simulink model "FullModel_Slow"  (R2024b)
settings: Solver=VariableStepAuto  StartTime=0.0  StopTime=50  FixedStep=1e-4  RelTol=1e-3  EnableMultiTasking=on
model workspace (MAT data in the model file):
  pidSample = 0.0005
  pwmFreq = 5000
libraries: nesl_utility x15, fl_lib x9, ee_lib x5, slpidlib x2, eeTransforms x1
settings Model: SimulationMode=accelerator  Creator=luigi  LastModifiedBy=luigi
settings SolverCC: AllowMultiTaskInputOutput=on  ConcurrentTasks=on  AutoInsertRateTranBlk=on  EnableFixedStepZeroCrossing=on
settings HardwareCC: ProdBitPerLong=64  ProdLargestAtomicFloat=None  ProdHWDeviceType=AMD->Athlon 64
settings SFSimCC: SimTargetLang=C++
settings RTWCC: RTWVerbose=off

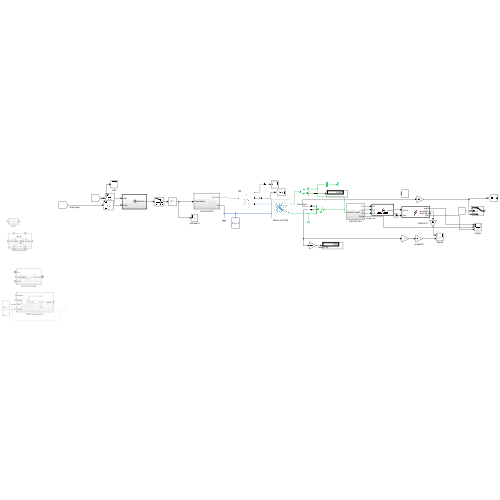
[thumbnail: Simulink's stored preview of the top-level diagram]
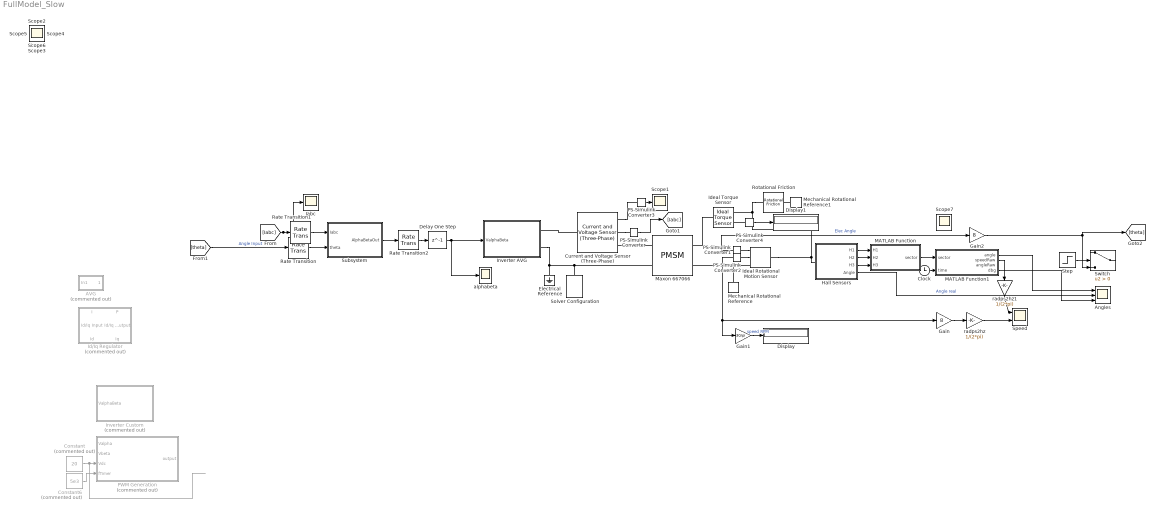
== system FullModel_Slow ==
  AVG : Subsystem  Commented=on
  Angles : Scope  NumInputPorts=3
  Clock : Clock
  Constant : Constant  Commented=on  Value=20
  Constant6 : Constant  Commented=on  Value=5e3
  Current and Voltage Sensor (Three-Phase) : ee_lib/Sensors & Transducers/Current and Voltage Sensor (Three-Phase)  vMeasurementType=ee.enum.vmeasurement.ll  outputUnit=ee.enum.unit.si  SRated=100e6 A*V  VRated=24e3 V  I_specify=off  I_priority=None  I=[0, 0, 0] A  I_nominal_specify=off  I_nominal_value=1  I_nominal_unit=A  V_specify=off  V_priority=None  V=[0, 0, 0] V  V_nominal_specify=off  V_nominal_value=1  V_nominal_unit=V
      settings: InternalSimscapePortConfiguration="{\"Bottom\":[],\"Left\":[{\"id\":\"N1\",\"label\":\"~1\",\"type\":\"foundation.electrical.three_phase\"}],\"Right\":[{\"id\":\"V_output\",\"label\":\"V\",\"type\":\"output\"},{\"id\":\"I_output\",\"label\":\"I\",\"type\":\"output\"},{\"id\":\"N2\",\"label\":\"~2\",\"type\":\"foundation.electrical.three_phase\"}],\"Top\":[]}"
  Delay One Step : Delay  DelayLength=1
  Display : Display
  Display1 : Display
  Electrical Reference : fl_lib/Electrical/Electrical Elements/Electrical Reference
  Gain : Gain  Gain=8
  Gain1 : Gain  Gain=30/pi
  Gain2 : Gain  Gain=8
  Hall Sensors : Subsystem
  Iabc : Scope
  Id/Iq Regulator : Subsystem  Commented=on
      settings: PortSchema="{\"entries\":[{\"content\":{\"sides\":[{\"content\":{\"connectorIds\":[\"In1\"]},\"type\":\"ConnectorPlacement.EquallySpacedRectSide\",\"uuid\":\"43b3a311-7cb7-4eab-a35c-85d0ca0e3076\"},{\"content\":{\"connectorIds\":[\"Out1\"],\"side\":\"RIGHT\"},\"type\":\"ConnectorPlacement.EquallySpacedRectSide\",\"uuid\":\"ca56bbca-54ba-4ca6-9209-c2819f440ab7\"},{\"content\":{\"connectorIds\":[\"In2\",\"In3\"],\"side\":\"TOP\"},\"type\":\"ConnectorPlacement.EquallySpacedRectSide\",\"uuid\":\"c57e1d45-56ff-40ef-8d87-b012e39b3f70\"},{\"content\":{\"connectorIds\":[\"In4\",\"In5\"],\"side\":\"BOTTOM\"},\"type\":\"ConnectorPlacement.EquallySpacedRectSide\",\"uuid\":\"5c883e63-5688-4569-9eaa-37faa042d8a8\"}]},\"type\":\"ConnectorPlacement.EquallySpacedConnector\",\"uuid\":\"9c051708-b157-4ef2-9fb2-e90e892a94b0\"}],\"packageUris\":[\"http://schema.mathworks.com/mf0/Connector/R2020b\"],\"version\":\"1.0\"}"
  Ideal Rotational Motion Sensor : fl_lib/Mechanical/Mechanical Sensors/Ideal Rotational Motion Sensor  reference=foundation.enum.MeasurementReference.difference  acceleration_port=false  velocity_port=true  position_port=true  wrap_angle=true  offset=0 rad
  Ideal Torque Sensor : fl_lib/Mechanical/Mechanical Sensors/Ideal Torque Sensor
  Inverter AVG : Subsystem
      settings: MinAlgLoopOccurrences=on
  Inverter Custom : Subsystem  Commented=on
      settings: PortSchema="{\"entries\":[{\"content\":{\"sides\":[{\"content\":{\"connectorIds\":[\"LConn1\",\"In1\",\"LConn2\"]},\"type\":\"ConnectorPlacement.EquallySpacedRectSide\",\"uuid\":\"8f29009c-fde7-40c5-b267-68669c6fe162\"},{\"content\":{\"connectorIds\":[\"RConn1\"],\"side\":\"RIGHT\"},\"type\":\"ConnectorPlacement.EquallySpacedRectSide\",\"uuid\":\"42ee2bc7-4e72-4e66-b818-79789fabddd4\"},{\"content\":{\"side\":\"TOP\"},\"type\":\"ConnectorPlacement.EquallySpacedRectSide\",\"uuid\":\"30675e7c-1db2-4723-9999-8a6d31f0d3a7\"}]},\"type\":\"ConnectorPlacement.EquallySpacedConnector\",\"uuid\":\"6307069a-32f5-4400-962e-81599f3d1bde\"}],\"packageUris\":[\"http://schema.mathworks.com/mf0/Connector/R2020b\"],\"version\":\"1.0\"}"
  MATLAB Function : MATLAB Function  TreatAsAtomicUnit=on  SystemSampleTime=0
  MATLAB Function1 : MATLAB Function  TreatAsAtomicUnit=on  SystemSampleTime=1e-4
  Maxon 667066 : ee_lib/Electromechanical/Permanent Magnet/PMSM  port_option=ee.enum.threePhasePort.composite  winding_type=ee.enum.electromech.statorconfiguration.wye  machine_param=ee.enum.pmsm.parameterization.constant  nPolePairs=8  pmflux_param=ee.enum.pmflux.torqueconstant  pm_flux_linkage=0.03 Wb  torque_constant=68 m*mN/A  back_emf_constant=0.18 V*s/rad  stator_param=ee.enum.statorparam.LsLmMs  Ld=0.00019 H  Lq=0.00025 H  idVec=[-200, 0, 200] A  iqVec=[-200, 0, 200] A  LdMatrix=0.0002 * ones(3, 3) H  LqMatrix=0.0002 * ones(3, 3) H  PmMatrix=0.1 * ones(3, 3) Wb  ktMatrix=0.18 * ones(3, 3) N*m/A  keMatrix=0.18 * ones(3, 3) V*s/rad  L0=0.00016 H  Ls=0.261/2 mH  Lm=0 H  Ms=0.261/4 mH  Rs=0.155/2 Ohm  zero_sequence=ee.enum.park.zerosequence.include  axes_param=ee.enum.rotorangle.daxis  loss_param=ee.enum.ironloss.none  losses_oc=[0, 0, 0] W  losses_sc=[0, 0, 0] W  f_losses=60 Hz  Isc_losses=95 A  J=0.01 kg*m^2  lam=0 N*m*s/rad  i_d_specify=off  i_d_priority=None  i_d=0 A  i_d_nominal_specify=off  i_d_nominal_value=1  i_d_nominal_unit=A  i_q_specify=off  i_q_priority=None  i_q=0 A  i_q_nominal_specify=off  i_q_nominal_value=1  i_q_nominal_unit=A  torque_specify=off  torque_priority=None  torque=0 N*m  torque_nominal_specify=off  torque_nominal_value=1  torque_nominal_unit=N*m  angular_velocity_specify=off  angular_velocity_priority=High  angular_velocity=500 rpm  angular_velocity_nominal_specify=off  angular_velocity_nominal_value=1  angular_velocity_nominal_unit=rpm  angular_position_specify=off  angular_position_priority=High  angular_position=0 deg  angular_position_nominal_specify=off  angular_position_nominal_value=1  angular_position_nominal_unit=deg  alpha=3.93e-3 1/K  alpha_flux=-0.001 1/K  Tmeas=298.15 K  stator_thermal_mass=100 J/K  rotor_thermal_mass=200 J/K  Rm_percent_rotor=90  Rd_percent_rotor=30  temperatureA_specify=off  temperatureA_priority=High  temperatureA=25 degC  temperatureA_nominal_specify=off  temperatureA_nominal_value=1  temperatureA_nominal_unit=degC  temperatureB_specify=off  temperatureB_priority=High  temperatureB=25 degC  temperatureB_nominal_specify=off  temperatureB_nominal_value=1  temperatureB_nominal_unit=degC  temperatureC_specify=off  temperatureC_priority=High  temperatureC=25 degC  temperatureC_nominal_specify=off  temperatureC_nominal_value=1  temperatureC_nominal_unit=degC  temperatureR_specify=off  temperatureR_priority=High  temperatureR=25 degC  temperatureR_nominal_specify=off  temperatureR_nominal_value=1  temperatureR_nominal_unit=degC
      settings: InternalSimscapePortConfiguration="{\"Bottom\":[],\"Left\":[{\"id\":\"N\",\"label\":\"~\",\"type\":\"foundation.electrical.three_phase\"},{\"id\":\"n\",\"label\":\"n\",\"type\":\"foundation.electrical.electrical\"}],\"Right\":[{\"id\":\"R\",\"label\":\"R\",\"type\":\"foundation.mechanical.rotational.rotational\"},{\"id\":\"C\",\"label\":\"C\",\"type\":\"foundation.mechanical.rotational.rotational\"}],\"Top\":[]}"
  Mechanical Rotational Reference : fl_lib/Mechanical/Rotational Elements/Mechanical Rotational Reference
  Mechanical Rotational Reference1 : fl_lib/Mechanical/Rotational Elements/Mechanical Rotational Reference
  PS-Simulink Converter{,1..4} (5 alike) : nesl_utility/PS-Simulink Converter  PhysicalDomain=network_engine_domain  SubClassName=ps_output  LeftPortType=input  RightPortType=output  PseudoPeriodic=off  Frequencies=[]  VectorFormat=inherit  Unit=inherit  AffineConversion=off
  PWM Generation : Subsystem  Commented=on
  Rate Transition : RateTransition
  Rate Transition1 : RateTransition
  Rate Transition2 : RateTransition
  Rotational Friction : fl_lib/Mechanical/Rotational Elements/Rotational Friction  brkwy_trq=0.1 N*m  brkwy_vel=0.1 rad/s  Col_trq=0.05 N*m  visc_coef=0.0005 N*m*s/rad  w_specify=off  w_priority=None  w=0 rad/s  w_nominal_specify=off  w_nominal_value=1  w_nominal_unit=rad/s  t_specify=off  t_priority=None  t=0 N*m  t_nominal_specify=off  t_nominal_value=1  t_nominal_unit=N*m
  Scope{,1..7} (8 alike) : Scope
  Solver Configuration : nesl_utility/Solver Configuration  PhysicalDomain=network_engine_domain  SubClassName=solver  LeftPortType=input  RightPortType=generic  Tones=[]  Harmonics=[]  SimulateNoise=off  Profile=off  UseLocalSampling=off  EnableSwitchedLinearOptims=on  FrequencyDomain=off  UseCCode=off  RelTol=0.001  AbsTol=0.001  MinStep=1e-09  ToWorkspace=off  RevertToSquareIcSolve=off  NumHomotopyIterations=100  PhasorMode=off  PhasorModeNumHarmonics=1  ConsistencySolver=NEWTON_XTOL_AFTER_FTOL  IndexReductionMethod=DerivativeReplacement  DoDC=off  ResidualTolerance=1e-09  ConsistencyTolSource=GLOBAL  ConsistencyAbsTol=0.001  ConsistencyRelTol=0.001  ConsistencyTolFactor=0.001  UseLocalSolver=on  LocalSolverChoice=NE_TRAPEZOIDAL_ADVANCER  ResolveIndetEquations=off  FunctionEvalNumThread=1  LocalSolverSampleTime=0.0001  DoFixedCost=off  MaxNonlinIter=3  MaxModeIter=2  ComputeImpulses=off  ImpulseIterations=2  LinearAlgebra=auto  LinearAlgebraNumThread=0  EquationFormulation=NE_TIME_EF  DelaysMemoryBudget=1024  AutomaticFiltering=off  FilteringTimeConstant=0.001  PartitionStorageMethod=AS_NEEDED  PartitionMemoryBudget=1024  PartitionMethod=ROBUST  MultibodyUseLocalSolver=off  MultibodyLocalSolverChoice=ODE1  MultibodyLocalSolverSampleTime=0.001
  Speed : Scope  NumInputPorts=2
  Step : Step  After=2  SampleTime=0
  Subsystem : Subsystem  TreatAsAtomicUnit=on  SystemSampleTime=1e-4
  Switch : Switch  Criteria=u2 > Threshold  SaturateOnIntegerOverflow=off  InputSameDT=off
  alphabeta : Scope
  radps2hz : Gain  Gain=1/(2*pi)
  radps2hz1 : Gain  Gain=1/(2*pi)
  wires:
  PS-Simulink Converter/1 -> [Iabc]
  Delay One Step/1 -> alphabeta/1, Inverter AVG/1(ValphaBeta)
  Hall Sensors/1(H1) -> MATLAB Function/1(H1)
  Hall Sensors/2(H2) -> MATLAB Function/2(H2)
  Hall Sensors/3(H3) -> MATLAB Function/3(H3)
  PS-Simulink Converter2/1 -> Gain1/1, Gain/1
  Constant/1 -> PWM Generation/3(Vdc)
  Constant6/1 -> PWM Generation/4(fTimer)
  PS-Simulink Converter3/1 -> Scope1/1
  Subsystem/1(AlphaBetaOut) -> Rate Transition2/1
  [Iabc] -> Iabc/1, Rate Transition1/1
  Rate Transition/1 -> Subsystem/2(theta)
  Rate Transition1/1 -> Subsystem/1(Iabc)
  Rate Transition2/1 -> Delay One Step/1
  [theta] -> Rate Transition/1  "Angle Input"
  Gain1/1 -> Display/1  "speed RPM"
  Step/1 -> Switch/2
  PS-Simulink Converter4/1 -> Display1/1
  PS-Simulink Converter1/1 -> Gain2/1  "Elec Angle"
  Gain2/1 -> Switch/3, [theta]
  MATLAB Function/1(sector) -> MATLAB Function1/1(sector)
  MATLAB Function1/2(speedRaw) -> radps2hz1/1
  MATLAB Function1/1(angle) -> Angles/1
  Hall Sensors/4(Angle) -> Angles/2  "Angle real"
  MATLAB Function1/4(dbg) -> Angles/3
  Clock/1 -> MATLAB Function1/2(time)
  Gain/1 -> radps2hz/1
  radps2hz/1 -> Speed/2
  radps2hz1/1 -> Speed/1
  connections:
  Solver Configuration/RConn1 -- Inverter AVG/RConn2 -- Electrical Reference/LConn1 -- Maxon 667066/LConn2
  Mechanical Rotational Reference/LConn1 -- Ideal Rotational Motion Sensor/RConn1 -- Maxon 667066/RConn2
  Current and Voltage Sensor (Three-Phase)/RConn3 -- Maxon 667066/LConn1
  PS-Simulink Converter1/LConn1 -- Ideal Rotational Motion Sensor/RConn3
  PS-Simulink Converter2/LConn1 -- Ideal Rotational Motion Sensor/RConn2
  Current and Voltage Sensor (Three-Phase)/RConn2 -- PS-Simulink Converter/LConn1
  Current and Voltage Sensor (Three-Phase)/RConn1 -- PS-Simulink Converter3/LConn1
  Current and Voltage Sensor (Three-Phase)/LConn1 -- Inverter AVG/RConn1
  Mechanical Rotational Reference1/LConn1 -- Rotational Friction/RConn1
  Rotational Friction/LConn1 -- Ideal Rotational Motion Sensor/LConn1 -- Hall Sensors/LConn1 -- Ideal Torque Sensor/RConn1
  Ideal Torque Sensor/LConn1 -- Maxon 667066/RConn1
  PS-Simulink Converter4/LConn1 -- Ideal Torque Sensor/RConn2

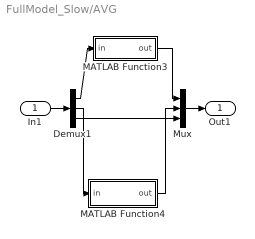
== system FullModel_Slow/AVG ==
  In1 : Inport
  Demux1 : Demux  Outputs=3
  MATLAB Function3 : MATLAB Function  TreatAsAtomicUnit=on  SystemSampleTime=0
  MATLAB Function4 : MATLAB Function  TreatAsAtomicUnit=on  SystemSampleTime=0
  Mux : Mux  Inputs=3
  Out1 : Outport
  wires:
  Demux1/1 -> MATLAB Function3/1(in)
  Demux1/2 -> MATLAB Function4/1(in)
  Demux1/3 -> Mux/3
  In1/1 -> Demux1/1
  MATLAB Function3/1(out) -> Mux/1
  MATLAB Function4/1(out) -> Mux/2
  Mux/1 -> Out1/1

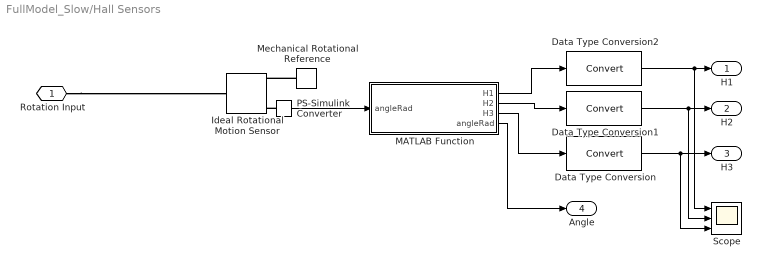
== system FullModel_Slow/Hall Sensors ==
  Data Type Conversion : DataTypeConversion  SaturateOnIntegerOverflow=off  RndMeth=Floor
  Data Type Conversion1 : DataTypeConversion  SaturateOnIntegerOverflow=off  RndMeth=Floor
  Data Type Conversion2 : DataTypeConversion  SaturateOnIntegerOverflow=off  RndMeth=Floor
  Ideal Rotational Motion Sensor : fl_lib/Mechanical/Mechanical Sensors/Ideal Rotational Motion Sensor  reference=foundation.enum.MeasurementReference.difference  acceleration_port=false  velocity_port=true  position_port=true  wrap_angle=true  offset=0 rad
  MATLAB Function : MATLAB Function  TreatAsAtomicUnit=on  SystemSampleTime=0
  Mechanical Rotational Reference : fl_lib/Mechanical/Rotational Elements/Mechanical Rotational Reference
  PS-Simulink Converter : nesl_utility/PS-Simulink Converter  PhysicalDomain=network_engine_domain  SubClassName=ps_output  LeftPortType=input  RightPortType=output  PseudoPeriodic=off  Frequencies=[]  VectorFormat=inherit  Unit=inherit  AffineConversion=off
  Scope : Scope  NumInputPorts=3
  Rotation Input : PMIOPort  Side=Left
  H1 : Outport  OutDataTypeStr=uint8
  H2 : Outport  Port=2  OutDataTypeStr=uint8
  H3 : Outport  Port=3  OutDataTypeStr=uint8
  Angle : Outport  Port=4  OutDataTypeStr=double
  wires:
  MATLAB Function/2(H2) -> Data Type Conversion1/1
  MATLAB Function/3(H3) -> Data Type Conversion/1
  PS-Simulink Converter/1 -> MATLAB Function/1("angleRad ")
  MATLAB Function/1(H1) -> Data Type Conversion2/1
  Data Type Conversion/1 -> Scope/3, H3/1
  Data Type Conversion1/1 -> Scope/2, H2/1
  Data Type Conversion2/1 -> H1/1, Scope/1
  MATLAB Function/4(angleRad) -> Angle/1
  connections:
  PS-Simulink Converter/LConn1 -- Ideal Rotational Motion Sensor/RConn3
  Mechanical Rotational Reference/LConn1 -- Ideal Rotational Motion Sensor/RConn1
  Rotation Input/RConn1 -- Ideal Rotational Motion Sensor/LConn1

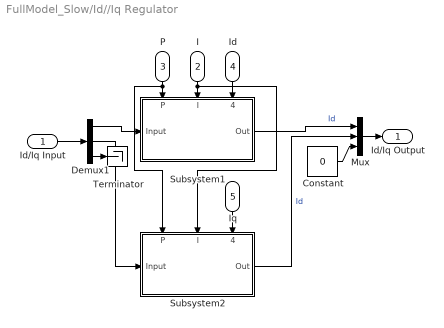
== system FullModel_Slow/Id//Iq Regulator ==
  Id/Iq Input : Inport
  I : Inport  Port=2
  P : Inport  Port=3
  Id : Inport  Port=4
  Iq : Inport  Port=5
  Constant : Constant  Value=0
  Demux1 : Demux  Outputs=3
  Mux : Mux  Inputs=3
  Subsystem1 : Subsystem
      settings: PortSchema="{\"entries\":[{\"content\":{\"sides\":[{\"content\":{\"connectorIds\":[\"In1\"]},\"type\":\"ConnectorPlacement.EquallySpacedRectSide\",\"uuid\":\"25e2072d-058f-4573-992d-939f168d4d75\"},{\"content\":{\"connectorIds\":[\"Out1\"],\"side\":\"RIGHT\"},\"type\":\"ConnectorPlacement.EquallySpacedRectSide\",\"uuid\":\"93949af7-0a35-4d0a-82f6-09dc0a159651\"},{\"content\":{\"connectorIds\":[\"In2\",\"In3\",\"In4\"],\"side\":\"TOP\"},\"type\":\"ConnectorPlacement.EquallySpacedRectSide\",\"uuid\":\"eea5aa7c-ee3c-40e1-b9f3-40dbe2d6b18b\"}]},\"type\":\"ConnectorPlacement.EquallySpacedConnector\",\"uuid\":\"a31f8809-a39f-4e5e-8d7a-4fb7b5627130\"}],\"packageUris\":[\"http://schema.mathworks.com/mf0/Connector/R2020b\"],\"version\":\"1.0\"}"
  Subsystem2 : Subsystem
      settings: PortSchema="{\"entries\":[{\"content\":{\"sides\":[{\"content\":{\"connectorIds\":[\"In1\"]},\"type\":\"ConnectorPlacement.EquallySpacedRectSide\",\"uuid\":\"25e2072d-058f-4573-992d-939f168d4d75\"},{\"content\":{\"connectorIds\":[\"Out1\"],\"side\":\"RIGHT\"},\"type\":\"ConnectorPlacement.EquallySpacedRectSide\",\"uuid\":\"93949af7-0a35-4d0a-82f6-09dc0a159651\"},{\"content\":{\"connectorIds\":[\"In2\",\"In3\",\"In4\"],\"side\":\"TOP\"},\"type\":\"ConnectorPlacement.EquallySpacedRectSide\",\"uuid\":\"eea5aa7c-ee3c-40e1-b9f3-40dbe2d6b18b\"}]},\"type\":\"ConnectorPlacement.EquallySpacedConnector\",\"uuid\":\"a31f8809-a39f-4e5e-8d7a-4fb7b5627130\"}],\"packageUris\":[\"http://schema.mathworks.com/mf0/Connector/R2020b\"],\"version\":\"1.0\"}"
  Terminator : Terminator
  Id/Iq Output : Outport
  wires:
  Id/Iq Input/1 -> Demux1/1
  P/1 -> Subsystem2/2(P), Subsystem1/2(P)
  Mux/1 -> Id/Iq Output/1
  I/1 -> Subsystem2/3(I), Subsystem1/3(I)
  Demux1/2 -> Subsystem2/1(Input)
  Iq/1 -> Subsystem2/4(Reference)
  Demux1/1 -> Subsystem1/1(Input)
  Id/1 -> Subsystem1/4(Reference)
  Subsystem1/1(Out) -> Mux/1  "Id"
  Demux1/3 -> Terminator/1
  Constant/1 -> Mux/3
  Subsystem2/1(Out) -> Mux/2  "Id"

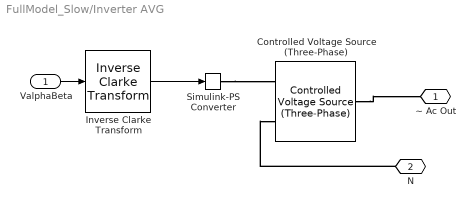
== system FullModel_Slow/Inverter AVG ==
  ValphaBeta : Inport
  Controlled Voltage Source (Three-Phase) : ee_lib/Sources/Controlled Voltage Source (Three-Phase)  input_option=ee.enum.inputType.instantaneous  FRated=60 Hz
      settings: InternalSimscapePortConfiguration="{\"Bottom\":[],\"Left\":[{\"id\":\"S\",\"label\":\"S\",\"type\":\"input\"},{\"id\":\"n\",\"label\":\"n\",\"type\":\"foundation.electrical.electrical\"}],\"Right\":[{\"id\":\"N\",\"label\":\"~\",\"type\":\"foundation.electrical.three_phase\"}],\"Top\":[]}"
  Inverse Clarke Transform : eeTransforms/Inverse Clarke Transform  PowerInvariant=off
  Simulink-PS Converter : nesl_utility/Simulink-PS Converter  PhysicalDomain=network_engine_domain  SubClassName=ps_input  LeftPortType=input  RightPortType=output  PseudoPeriodic=off  Frequencies=[]  NoiseDistribution=none  NoiseParameters=[]  Unit=1  AffineConversion=off  FilteringAndDerivatives=provide  SimscapeFilterOrder=1  InputFilterTimeConstant=0.001  UdotUserProvided=0
  ~ Ac Out : PMIOPort  Side=Right
  N : PMIOPort  Port=2  Side=Right
  wires:
  ValphaBeta/1 -> Inverse Clarke Transform/1
  Inverse Clarke Transform/1 -> Simulink-PS Converter/1
  connections:
  Controlled Voltage Source (Three-Phase)/RConn1 -- ~ Ac Out/RConn1
  Simulink-PS Converter/RConn1 -- Controlled Voltage Source (Three-Phase)/LConn1
  N/RConn1 -- Controlled Voltage Source (Three-Phase)/LConn2

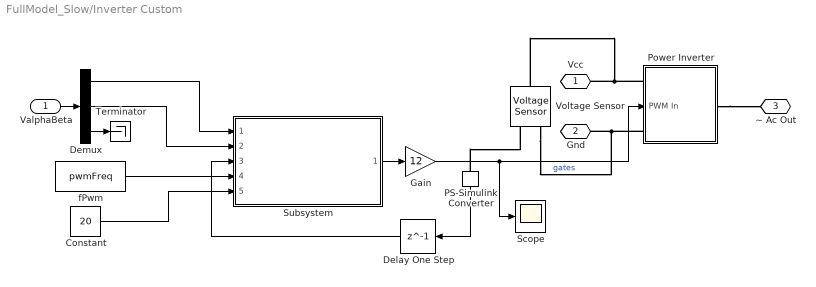
== system FullModel_Slow/Inverter Custom ==
  ValphaBeta : Inport
  Constant : Constant  Value=20
  Delay One Step : Delay  DelayLength=1
  Demux : Demux  Outputs=3
  Gain : Gain  Gain=12
  PS-Simulink Converter : nesl_utility/PS-Simulink Converter  PhysicalDomain=network_engine_domain  SubClassName=ps_output  LeftPortType=input  RightPortType=output  PseudoPeriodic=off  Frequencies=[]  VectorFormat=inherit  Unit=inherit  AffineConversion=off
  Power Inverter : Subsystem
      settings: PortSchema="{\"entries\":[{\"content\":{\"sides\":[{\"content\":{\"connectorIds\":[\"LConn1\"]},\"type\":\"ConnectorPlacement.EquallySpacedRectSide\",\"uuid\":\"8f29009c-fde7-40c5-b267-68669c6fe162\"},{\"content\":{\"connectorIds\":[\"RConn1\",\"In1\",\"RConn2\"],\"side\":\"RIGHT\"},\"type\":\"ConnectorPlacement.EquallySpacedRectSide\",\"uuid\":\"42ee2bc7-4e72-4e66-b818-79789fabddd4\"},{\"content\":{\"side\":\"TOP\"},\"type\":\"ConnectorPlacement.EquallySpacedRectSide\",\"uuid\":\"30675e7c-1db2-4723-9999-8a6d31f0d3a7\"}]},\"type\":\"ConnectorPlacement.EquallySpacedConnector\",\"uuid\":\"6307069a-32f5-4400-962e-81599f3d1bde\"}],\"packageUris\":[\"http://schema.mathworks.com/mf0/Connector/R2020b\"],\"version\":\"1.0\"}"
  Scope : Scope
  Subsystem : Subsystem  TreatAsAtomicUnit=on  SystemSampleTime=0.1/pwmFreq  ReferencedSubsystem=InverterLogic
  Terminator : Terminator
  Voltage Sensor : fl_lib/Electrical/Electrical Sensors/Voltage Sensor
  fPwm : Constant  Value=pwmFreq
  Vcc : PMIOPort  Side=Left
  Gnd : PMIOPort  Port=2  Side=Left
  ~ Ac Out : PMIOPort  Port=3  Side=Right
  wires:
  ValphaBeta/1 -> Demux/1
  Demux/3 -> Terminator/1
  Demux/1 -> Subsystem/1
  Demux/2 -> Subsystem/2
  PS-Simulink Converter/1 -> Delay One Step/1
  fPwm/1 -> Subsystem/4
  Constant/1 -> Subsystem/5
  Subsystem/1 -> Gain/1
  Gain/1 -> Scope/1, Power Inverter/1(PWM In)  "gates"
  Delay One Step/1 -> Subsystem/3
  connections:
  Power Inverter/RConn2 -- Voltage Sensor/RConn2 -- Gnd/RConn1
  Power Inverter/RConn1 -- Voltage Sensor/LConn1 -- Vcc/RConn1
  Power Inverter/LConn1 -- ~ Ac Out/RConn1
  PS-Simulink Converter/LConn1 -- Voltage Sensor/RConn1

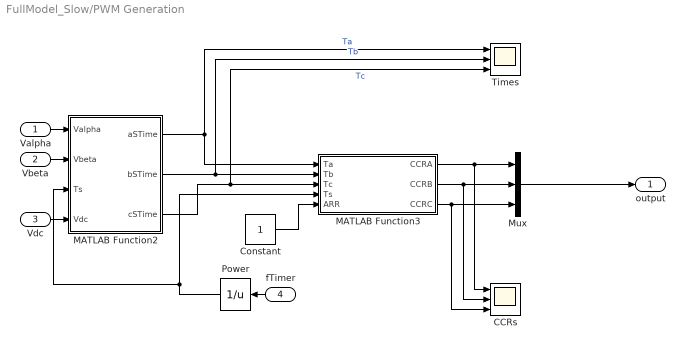
== system FullModel_Slow/PWM Generation ==
  Valpha : Inport
  Vbeta : Inport  Port=2
  Vdc : Inport  Port=3
  fTimer : Inport  Port=4
  CCRs : Scope  NumInputPorts=3
  Constant : Constant
  MATLAB Function2 : MATLAB Function  TreatAsAtomicUnit=on
  MATLAB Function3 : MATLAB Function  TreatAsAtomicUnit=on
  Mux : Mux  Inputs=3
  Power : Math  Operator=reciprocal
  Times : Scope  NumInputPorts=3
  output : Outport
  wires:
  Valpha/1 -> MATLAB Function2/1(Valpha)
  Vdc/1 -> MATLAB Function2/4(Vdc)
  MATLAB Function2/1(aSTime) -> MATLAB Function3/1(Ta), Times/1  "Ta"
  MATLAB Function2/3(cSTime) -> Times/3, MATLAB Function3/3(Tc)  "Tc"
  Power/1 -> MATLAB Function2/3(Ts), MATLAB Function3/4(Ts)
  Vbeta/1 -> MATLAB Function2/2(Vbeta)
  MATLAB Function2/2(bSTime) -> Times/2, MATLAB Function3/2(Tb)  "Tb"
  MATLAB Function3/1(CCRA) -> Mux/1, CCRs/1
  Mux/1 -> output/1
  MATLAB Function3/3(CCRC) -> Mux/3, CCRs/3
  MATLAB Function3/2(CCRB) -> Mux/2, CCRs/2
  fTimer/1 -> Power/1
  Constant/1 -> MATLAB Function3/5(ARR)

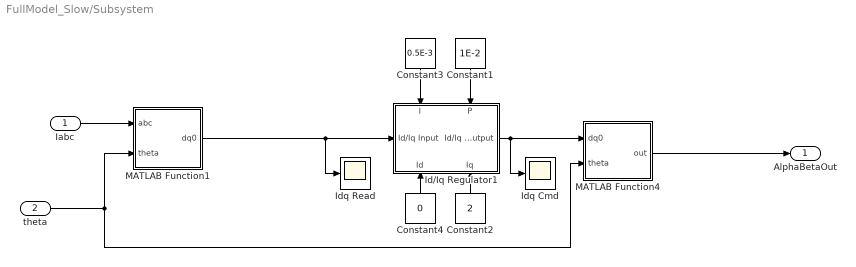
== system FullModel_Slow/Subsystem ==
  Iabc : Inport
  theta : Inport  Port=2
  Constant1 : Constant  Value=1E-2
  Constant2 : Constant  Value=2
  Constant3 : Constant  Value=0.5E-3
  Constant4 : Constant  Value=0
  Id/Iq Regulator1 : Subsystem  TreatAsAtomicUnit=on
      settings: PortSchema="{\"entries\":[{\"content\":{\"sides\":[{\"content\":{\"connectorIds\":[\"In1\"]},\"type\":\"ConnectorPlacement.EquallySpacedRectSide\",\"uuid\":\"43b3a311-7cb7-4eab-a35c-85d0ca0e3076\"},{\"content\":{\"connectorIds\":[\"Out1\"],\"side\":\"RIGHT\"},\"type\":\"ConnectorPlacement.EquallySpacedRectSide\",\"uuid\":\"ca56bbca-54ba-4ca6-9209-c2819f440ab7\"},{\"content\":{\"connectorIds\":[\"In2\",\"In3\"],\"side\":\"TOP\"},\"type\":\"ConnectorPlacement.EquallySpacedRectSide\",\"uuid\":\"c57e1d45-56ff-40ef-8d87-b012e39b3f70\"},{\"content\":{\"connectorIds\":[\"In4\",\"In5\"],\"side\":\"BOTTOM\"},\"type\":\"ConnectorPlacement.EquallySpacedRectSide\",\"uuid\":\"5c883e63-5688-4569-9eaa-37faa042d8a8\"}]},\"type\":\"ConnectorPlacement.EquallySpacedConnector\",\"uuid\":\"9c051708-b157-4ef2-9fb2-e90e892a94b0\"}],\"packageUris\":[\"http://schema.mathworks.com/mf0/Connector/R2020b\"],\"version\":\"1.0\"}"
  Idq Cmd : Scope
  Idq Read : Scope
  MATLAB Function1 : MATLAB Function  TreatAsAtomicUnit=on
  MATLAB Function4 : MATLAB Function  TreatAsAtomicUnit=on
  AlphaBetaOut : Outport
  wires:
  MATLAB Function4/1(out) -> AlphaBetaOut/1
  Constant3/1 -> Id/Iq Regulator1/2(I)
  Constant2/1 -> Id/Iq Regulator1/5(Iq)
  Iabc/1 -> MATLAB Function1/1(abc)
  Constant4/1 -> Id/Iq Regulator1/4(Id)
  theta/1 -> MATLAB Function1/2(theta), MATLAB Function4/2(theta)
  Constant1/1 -> Id/Iq Regulator1/3(P)
  MATLAB Function1/1(dq0) -> Id/Iq Regulator1/1(Id/Iq Input), Idq Read/1
  Id/Iq Regulator1/1(Id/Iq Output) -> MATLAB Function4/1(dq0), Idq Cmd/1

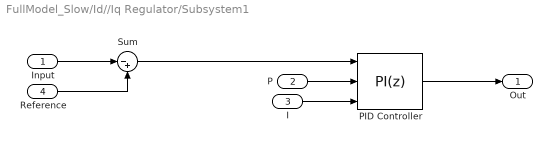
== system FullModel_Slow/Id//Iq Regulator/Subsystem1 ==
  Input : Inport
  P : Inport  Port=2
  I : Inport  Port=3
  Reference : Inport  Port=4
  PID Controller : slpidlib/PID Controller  Controller=PI  Form=Parallel  TimeDomain=Discrete-time  UseExternalTs=off  SampleTime=-1  IntegratorMethod=Forward Euler  FilterMethod=Forward Euler  ControllerParametersSource=external  P=0.068581  I=0  UseKiTs=off  D=0  UseExternalDerivativeSource=off  N=100  UseFilter=on  TunerSelectOption=Frequency Response Based  InitialConditionSource=internal  InitialConditionForIntegrator=0  InitialConditionForFilter=0  DifferentiatorICPrevScaledInput=0  ExternalReset=none  TrackingMode=off  Kt=1  LimitOutput=off  SatLimitsSource=internal  UpperSaturationLimit=inf  LowerSaturationLimit=-inf  LinearizeAsGain=on  AntiWindupMode=none  Kb=1  LimitIntegrator=off  UpperIntegratorSaturationLimit=inf  LowerIntegratorSaturationLimit=-inf  POutMin=[]  POutMax=[]  IOutMin=[]  IOutMax=[]  DOutMin=[]  DOutMax=[]  NOutMin=[]  NOutMax=[]  SumOutMin=[]  SumOutMax=[]  SaturationOutMin=[]  SaturationOutMax=[]  PParamMin=[]  PParamMax=[]  IParamMin=[]  IParamMax=[]  DParamMin=[]  DParamMax=[]  NParamMin=[]  NParamMax=[]  KbParamMin=[]  KbParamMax=[]  KtParamMin=[]  KtParamMax=[]  KbOutMin=[]  KbOutMax=[]  KtOutMin=[]  KtOutMax=[]  IntegratorOutMin=[]  IntegratorOutMax=[]  FilterOutMin=[]  FilterOutMax=[]  SumI1OutMin=[]  SumI1OutMax=[]  SumI2OutMin=[]  SumI2OutMax=[]  SumI3OutMin=[]  SumI3OutMax=[]  SumI4OutMin=[]  SumI4OutMax=[]  SumDOutMin=[]  SumDOutMax=[]  DifferentiatorOutMin=[]  DifferentiatorOutMax=[]  FilterDiffOutCoefMin=[]  FilterDiffOutCoefMax=[]  ReciprocalOutMin=[]  ReciprocalOutMax=[]  SumDenOutMin=[]  SumDenOutMax=[]  SumNumOutMin=[]  SumNumOutMax=[]  DivideOutMin=[]  DivideOutMax=[]  UdiffTsProdOutMin=[]  UdiffTsProdOutMax=[]  NTsProdOutMin=[]  NTsProdOutMax=[]  UintegralTsProdOutMin=[]  UintegralTsProdOutMax=[]  UngainTsProdOutMin=[]  UngainTsProdOutMax=[]  ClampingZeroOutDataTypeStr=Inherit: Inherit via back propagation  ClampingZeroOutMin=[]  ClampingZeroOutMax=[]  FilterDenConstantOutDataTypeStr=Inherit: Inherit via back propagation  FilterDenConstantOutMin=[]  FilterDenConstantOutMax=[]  PCopyOutDataTypeStr=Inherit: Inherit via back propagation  PCopyOutMin=[]  PCopyOutMax=[]  NCopyOutDataTypeStr=Inherit: Inherit via back propagation  NCopyOutMin=[]  NCopyOutMax=[]  IntegratorContinuousStateAttributes=''  IntegratorStateMustResolveToSignalObject=off  IntegratorRTWStateStorageClass=Auto  FilterContinuousStateAttributes=''  FilterStateMustResolveToSignalObject=off  FilterRTWStateStorageClass=Auto  ParallelPVariant=ExternalParameters  IdealPVariant=Disabled  IVariant=ExternalParameters  DVariant=Disabled  IntegratorVariant=Discrete  SatVariant=Disabled  AWVariant=Passthrough  PCopyVariant=Disabled  TRVariant=Disabled  FdbkBlocksVariant=Forward  IdealPFdbkVariant=Disabled  SatFdbkVariant=Disabled  DerivativeFilterVariant=Disabled  NVariant=Disabled  NCopyVariant=Disabled_SignalSpec  FilterICVariant=Disabled  IntegratorICVariant=InternalICs  ExternalResetVariant=Disabled  TRSumVariant=Passthrough  SumFdbkVariant=Disabled  SumVariant=Sum_PI  TsampFilterVariant=InternalTs  TsampNgainVariant=Passthrough  TsampIntegralVariant=Disabled_SignalSpec  ExternalSaturationOutDataTypeStr=Inherit: Same as second input  DerivativeSourceVariant=Disabled  PreIntVariant=InternalPreInt
  Sum : Sum  Inputs=|-+
  Out : Outport
  wires:
  P/1 -> PID Controller/2
  Reference/1 -> Sum/2
  I/1 -> PID Controller/3
  Input/1 -> Sum/1
  PID Controller/1 -> Out/1
  Sum/1 -> PID Controller/1

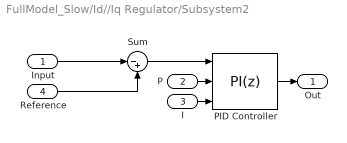
== system FullModel_Slow/Id//Iq Regulator/Subsystem2 ==
  Input : Inport
  P : Inport  Port=2
  I : Inport  Port=3
  Reference : Inport  Port=4
  PID Controller : slpidlib/PID Controller  Controller=PI  Form=Parallel  TimeDomain=Discrete-time  UseExternalTs=off  SampleTime=-1  IntegratorMethod=Forward Euler  FilterMethod=Forward Euler  ControllerParametersSource=external  P=1  I=1  UseKiTs=off  D=0  UseExternalDerivativeSource=off  N=100  UseFilter=on  TunerSelectOption=Transfer Function Based (PID Tuner App)  InitialConditionSource=internal  InitialConditionForIntegrator=0  InitialConditionForFilter=0  DifferentiatorICPrevScaledInput=0  ExternalReset=none  TrackingMode=off  Kt=1  LimitOutput=off  SatLimitsSource=internal  UpperSaturationLimit=inf  LowerSaturationLimit=-inf  LinearizeAsGain=on  AntiWindupMode=none  Kb=1  LimitIntegrator=off  UpperIntegratorSaturationLimit=inf  LowerIntegratorSaturationLimit=-inf  POutMin=[]  POutMax=[]  IOutMin=[]  IOutMax=[]  DOutMin=[]  DOutMax=[]  NOutMin=[]  NOutMax=[]  SumOutMin=[]  SumOutMax=[]  SaturationOutMin=[]  SaturationOutMax=[]  PParamMin=[]  PParamMax=[]  IParamMin=[]  IParamMax=[]  DParamMin=[]  DParamMax=[]  NParamMin=[]  NParamMax=[]  KbParamMin=[]  KbParamMax=[]  KtParamMin=[]  KtParamMax=[]  KbOutMin=[]  KbOutMax=[]  KtOutMin=[]  KtOutMax=[]  IntegratorOutMin=[]  IntegratorOutMax=[]  FilterOutMin=[]  FilterOutMax=[]  SumI1OutMin=[]  SumI1OutMax=[]  SumI2OutMin=[]  SumI2OutMax=[]  SumI3OutMin=[]  SumI3OutMax=[]  SumI4OutMin=[]  SumI4OutMax=[]  SumDOutMin=[]  SumDOutMax=[]  DifferentiatorOutMin=[]  DifferentiatorOutMax=[]  FilterDiffOutCoefMin=[]  FilterDiffOutCoefMax=[]  ReciprocalOutMin=[]  ReciprocalOutMax=[]  SumDenOutMin=[]  SumDenOutMax=[]  SumNumOutMin=[]  SumNumOutMax=[]  DivideOutMin=[]  DivideOutMax=[]  UdiffTsProdOutMin=[]  UdiffTsProdOutMax=[]  NTsProdOutMin=[]  NTsProdOutMax=[]  UintegralTsProdOutMin=[]  UintegralTsProdOutMax=[]  UngainTsProdOutMin=[]  UngainTsProdOutMax=[]  ClampingZeroOutDataTypeStr=Inherit: Inherit via back propagation  ClampingZeroOutMin=[]  ClampingZeroOutMax=[]  FilterDenConstantOutDataTypeStr=Inherit: Inherit via back propagation  FilterDenConstantOutMin=[]  FilterDenConstantOutMax=[]  PCopyOutDataTypeStr=Inherit: Inherit via back propagation  PCopyOutMin=[]  PCopyOutMax=[]  NCopyOutDataTypeStr=Inherit: Inherit via back propagation  NCopyOutMin=[]  NCopyOutMax=[]  IntegratorContinuousStateAttributes=''  IntegratorStateMustResolveToSignalObject=off  IntegratorRTWStateStorageClass=Auto  FilterContinuousStateAttributes=''  FilterStateMustResolveToSignalObject=off  FilterRTWStateStorageClass=Auto  ParallelPVariant=ExternalParameters  IdealPVariant=Disabled  IVariant=ExternalParameters  DVariant=Disabled  IntegratorVariant=Discrete  SatVariant=Disabled  AWVariant=Passthrough  PCopyVariant=Disabled  TRVariant=Disabled  FdbkBlocksVariant=Forward  IdealPFdbkVariant=Disabled  SatFdbkVariant=Disabled  DerivativeFilterVariant=Disabled  NVariant=Disabled  NCopyVariant=Disabled_SignalSpec  FilterICVariant=Disabled  IntegratorICVariant=InternalICs  ExternalResetVariant=Disabled  TRSumVariant=Passthrough  SumFdbkVariant=Disabled  SumVariant=Sum_PI  TsampFilterVariant=InternalTs  TsampNgainVariant=Passthrough  TsampIntegralVariant=Disabled_SignalSpec  ExternalSaturationOutDataTypeStr=Inherit: Same as second input  DerivativeSourceVariant=Disabled  PreIntVariant=InternalPreInt
  Sum : Sum  Inputs=|-+
  Out : Outport
  wires:
  Sum/1 -> PID Controller/1
  P/1 -> PID Controller/2
  PID Controller/1 -> Out/1
  Reference/1 -> Sum/2
  I/1 -> PID Controller/3
  Input/1 -> Sum/1

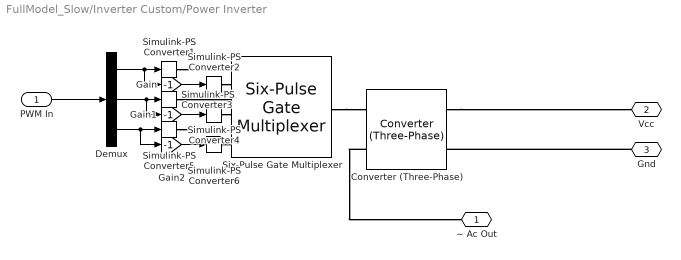
== system FullModel_Slow/Inverter Custom/Power Inverter ==
  PWM In : Inport
  Converter (Three-Phase) : ee_lib/Semiconductors & Converters/Converters/Converter (Three-Phase)  port_option=ee.enum.threePhasePort.composite  fidelity_option=ee.enum.converters.fidelity.detailed  device_type=ee.enum.converters.switchingdevice.ideal  showThermalPort=false  K=0  Vth=6 V  Vgt=1 V  Vgt_off=-1 V  Ih=1 A  Vf=0.8 V  Ron=0.001 Ohm  Rds=0.001 Ohm  Goff=1e-6 1/Ohm  Eon_scalar=22.86e-3 J  Eoff_scalar=17.14e-3 J  Eoff_natural_commutation=10e-3 J  Voff=300 V  Iout_scalar=600 A  onCurrentMeasDelay=0 s  useCurrentFromPreviousCycle=false  useVoltageFromPreviousCycle=false  diode_param=ee.enum.converters.protectiondiode.none  diode_Vf=0.8 V  diode_Ron=0.001 Ohm  diode_Goff=1e-5 1/Ohm  diode_C=50 nF  diode_iRM=-235 A  diode_iF=300 A  diode_idot=-50 A/us  diode_trr_param=ee.enum.converters.diodetrr.trr_factor  diode_trr_factor=3  diode_trr=15 us  diode_Qrr=1500 s*uA  diode_rec_loss_model=ee.enum.diode.reverseRecoveryModel.fixed  diode_ErecVal=0 J  diode_scaleWithIandV=false  diode_ErecMat=zeros(2, 3) J  diode_TjrecVec=[298.15, 398.15] K  diode_IfrecVec=[.1, 1, 10] A  diode_IrecVal=10 A  diode_VrecVal=10 V  diode_tFilter=1 / 1000 / 100 s  thermal_network_parameterization=ee.enum.thermalNetworkTopology.external  Rth=[.08, .5] K/W  Rth_Cauer=[.08, .1, .5] K/W  Rth_Foster=[.08, .14, .22, .16] K/W  thermal_mass_parameterization=ee.enum.thermalNetwork.timeconstant  thermal_mass=[.01, .5] J/K  thermal_mass_Cauer=[.01, .1, .5] J/K  thermal_mass_Foster=[.001, .005, .05, .5] J/K  thermal_time_constant=[.001, .2] s  thermal_time_constant_Cauer=[.001, .1, .2] s  thermal_time_constant_Foster=[7e-05, .0007, .01, .08] s  thermal_mass_initial_temperatures=[25, 25] degC  thermal_mass_initial_temperatures_Cauer=[25, 25, 25] degC  junction_thermal_mass=0.01 J/K  Tvec_initial_Foster=[25, 25, 25, 25] degC  snubber_type=ee.enum.converters.snubber.exclude  Cs=1e-7 F  Rs=0.1 Ohm  Vce_loss=[0, 150, 300] V
  Demux : Demux  Outputs=3
  Gain : Gain  Gain=-1
  Gain1 : Gain  Gain=-1
  Gain2 : Gain  Gain=-1
  Simulink-PS Converter{1..6} (6 alike) : nesl_utility/Simulink-PS Converter  PhysicalDomain=network_engine_domain  SubClassName=ps_input  LeftPortType=input  RightPortType=output  PseudoPeriodic=off  Frequencies=[]  NoiseDistribution=none  NoiseParameters=[]  Unit=1  AffineConversion=off  FilteringAndDerivatives=provide  SimscapeFilterOrder=1  InputFilterTimeConstant=0.001  UdotUserProvided=0
  Six-Pulse Gate Multiplexer : ee_lib/Semiconductors & Converters/Converters/Six-Pulse Gate Multiplexer  port_option=ee.enum.controlport.ps
  ~ Ac Out : PMIOPort  Side=Left
  Vcc : PMIOPort  Port=2  Side=Right
  Gnd : PMIOPort  Port=3  Side=Right
  wires:
  PWM In/1 -> Demux/1
  Demux/3 -> Gain2/1, Simulink-PS Converter5/1
  Demux/2 -> Gain1/1, Simulink-PS Converter3/1
  Demux/1 -> Gain/1, Simulink-PS Converter1/1
  Gain/1 -> Simulink-PS Converter2/1
  Gain1/1 -> Simulink-PS Converter4/1
  Gain2/1 -> Simulink-PS Converter6/1
  connections:
  Simulink-PS Converter3/RConn1 -- Six-Pulse Gate Multiplexer/LConn3
  Simulink-PS Converter6/RConn1 -- Six-Pulse Gate Multiplexer/LConn6
  Simulink-PS Converter1/RConn1 -- Six-Pulse Gate Multiplexer/LConn1
  Simulink-PS Converter4/RConn1 -- Six-Pulse Gate Multiplexer/LConn4
  Converter (Three-Phase)/RConn1 -- Vcc/RConn1
  Gnd/RConn1 -- Converter (Three-Phase)/RConn2
  Converter (Three-Phase)/LConn2 -- ~ Ac Out/RConn1
  Six-Pulse Gate Multiplexer/RConn1 -- Converter (Three-Phase)/LConn1
  Simulink-PS Converter5/RConn1 -- Six-Pulse Gate Multiplexer/LConn5
  Simulink-PS Converter2/RConn1 -- Six-Pulse Gate Multiplexer/LConn2

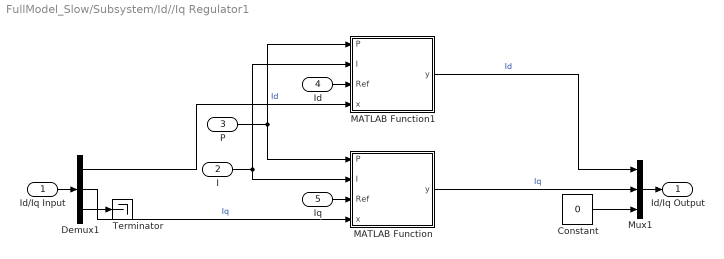
== system FullModel_Slow/Subsystem/Id//Iq Regulator1 ==
  Id/Iq Input : Inport
  I : Inport  Port=2
  P : Inport  Port=3
  Id : Inport  Port=4
  Iq : Inport  Port=5
  Constant : Constant  Value=0
  Demux1 : Demux  Outputs=3
  MATLAB Function : MATLAB Function  TreatAsAtomicUnit=on
  MATLAB Function1 : MATLAB Function  TreatAsAtomicUnit=on
  Mux1 : Mux  Inputs=3
  Terminator : Terminator
  Id/Iq Output : Outport
  wires:
  MATLAB Function1/1(y) -> Mux1/1  "Id"
  Id/Iq Input/1 -> Demux1/1
  P/1 -> MATLAB Function1/1(P), MATLAB Function/1(P)
  Demux1/1 -> MATLAB Function1/4(x)  "Id"
  MATLAB Function/1(y) -> Mux1/2  "Iq"
  Mux1/1 -> Id/Iq Output/1
  Demux1/2 -> MATLAB Function/4(x)  "Iq"
  I/1 -> MATLAB Function/2(I), MATLAB Function1/2(I)
  Demux1/3 -> Terminator/1
  Constant/1 -> Mux1/3
  Iq/1 -> MATLAB Function/3(Ref)
  Id/1 -> MATLAB Function1/3(Ref)

== matlab function FullModel_Slow/MATLAB Function ==
  data: H1 input; sector output; H2 input; H3 input
function sector = getSector(H1,H2,H3)

positionIndex = bitor(H1, bitor(bitshift(H2, 1), bitshift(H3, 2)));
sector = -1;
switch positionIndex
    case 0b101
        sector = 0;
    case 0b100
        sector = 0;
    case 0b110
        sector = 4;
    case 0b010
        sector = 4;
    case 0b011
        sector = 2;
    case 0b001
        sector = 2;
   
end

== matlab function FullModel_Slow/MATLAB Function1 ==
  data: sector input; angle output; time input; speedRaw output; angleRaw output; dbg output
function [angle, speedRaw, angleRaw, dbg] = fcn(sector, time)

DELTA_ANGLE_RAD = pi/3;

SPEED_AVG = 10;


% dbg = -1;
persistent oldSector
if isempty(oldSector)
    oldSector = 0;
end
persistent oldTime
if isempty(oldTime)
    oldTime = 0;
end
persistent oldRTime
if isempty(oldRTime)
    oldRTime = 0;
end
persistent speed
if isempty(speed)
    speed = 0;
end
persistent prevAngle
if isempty(prevAngle)
    prevAngle = rand(1) * 2*pi;
end
persistent oldDir
if isempty(oldDir)
    oldDir = 0;
end
persistent errorIntegral
if isempty(errorIntegral)
    errorIntegral = 0;
end
persistent revCountMeas
if isempty(revCountMeas)
    revCountMeas = 0;
end
persistent revCountOut
if isempty(revCountOut)
    revCountOut = 0;
end
persistent angleError
if isempty(angleError)
    angleError = 0;
end

angleRaw = sector * DELTA_ANGLE_RAD;
if(sector ~= oldSector)
    dT = time - oldTime;
    
    if(sector == 0)
        revCountMeas = revCountMeas + 1;
    end

    %Direction detection and maintaining 
    % dSector = oldSector - sector;
    % 
    % if dSector > 3
    %     newDir = -1;
    % elseif dSector < -3
    %     newDir = 1;
    % elseif sector > oldSector
    %     newDir = -1;
    % else 
    %     newDir = 1;
    % end
    % 
    % if oldDir ~= 0
    %     if oldDir ~= newDir
    %         prevAngle = -1;
    %     end
    % else
    %     oldDir = newDir;
    % end
    % Speed, and phase locking
    
    % angleError = 2*pi*(revCountMeas - revCountOut) + angleRaw - prevAngle;
    angleError = angleRaw - prevAngle;
   
    % if angleError > pi
    %     angleError = angleError - 2*pi;
    % elseif angleError < -pi
    %     angleError = angleError + 2*pi;
    % end
    
    if dT > 0
        speedTmp = 2*DELTA_ANGLE_RAD / dT; % Basic speed compute
        if oldDir == 0
         prevAngle = angleRaw;
         oldDir = 1;
        end
        % speedTmp = speedTmp + errorIntegral * 2; % Integral term
        % speedTmp = speedTmp + angleError * 0.5; % Proportional term
        
        speed = speed - speed / SPEED_AVG;
        speed = speed + speedTmp / SPEED_AVG;
    end
    oldTime = time;
    oldSector = sector;
    errorIntegral = 0;
end

errorIntegral = errorIntegral + angleError * (time - oldRTime);

errorSim = rand(1); % Produces from 0 to 1 perccent  error

prevAngle = prevAngle + speed * (time - oldRTime);
oldRTime = time;

if prevAngle > 2*pi
    prevAngle = prevAngle - 2*pi;
    revCountOut = revCountOut + 1;
elseif prevAngle < -2*pi
    prevAngle = prevAngle + 2*pi;
    revCountOut = revCountOut + 1;
end
dbg = errorIntegral;
angle = prevAngle ;
speedRaw = speed;

== matlab function FullModel_Slow/Subsystem/MATLAB Function1 ==
  data: abc input; theta input; dq0 output
function dq0 = parkTf(abc, theta)
dq0 = zeros(3, 1);
cosine = cos(theta);
sine = sin(theta);

alpha = abc(1);
beta = abc(1) * (1./sqrt(3)) + abc(2) * (2./sqrt(3));

% D aligned
dq0(1) = alpha * cosine + beta * sine;
dq0(2) = - alpha * sine + beta * cosine;
dq0(3) = 0;

% Q aligned
% dq0(1) = alpha * sine - beta * cosine;
% dq0(2) = alpha * cosine + beta * sine;
% dq0(3) = 0;

== matlab function FullModel_Slow/PWM Generation/MATLAB Function2 ==
  data: Valpha input; aSTime output; Vbeta input; Ts input; Vdc input; bSTime output; cSTime output
function [aSTime, bSTime, cSTime] = SVPWM(Valpha, Vbeta, Ts, Vdc)
Ts = Ts./2;

piThird = pi/3;
scaling = 2/sqrt(3);


% First step: determine the angle of the reference
if(Valpha == 0)
    theta = 0;
else
    theta = atan(Vbeta/Valpha);
end

if(theta < 0)
    theta = theta + pi;
end

if(Vbeta < 0)
    theta = theta + pi;
end

Vref = sqrt(Valpha*Valpha+Vbeta*Vbeta);

quad = floor(theta/piThird) + 1;

modulation = (3/2) * (Vref/Vdc);

ThB = (quad-1) * piThird; %Angle of first possible vector
ThA = quad * piThird; %Angle of the second vector

Ta = scaling * modulation * Ts * sin(ThA - theta);
Tb = scaling * modulation * Ts * sin(theta - ThB);
Tz = Ts - Ta - Tb;

aSTime = 0;
bSTime = 0;
cSTime = 0;

switch quad
    case 1
        aSTime = Ta + Tb + Tz/2;
        bSTime = Tb + Tz/2;
        cSTime = Tz/2;
    case 2
        aSTime = Ta + Tz/2;
        bSTime  = Ta + Tb + Tz/2;
        cSTime  = Tz/2;
    case 3
        aSTime = Tz/2;
        bSTime = Ta + Tb + Tz/2;
        cSTime  = Tb + Tz/2;
    case 4
        aSTime = Tz/2;
        bSTime = Ta + Tz/2;
        cSTime  = Ta + Tb + Tz/2;
    case 5
        aSTime = Tb + Tz/2;
        bSTime = Tz/2;
        cSTime = Ta + Tb + Tz/2;
    case 6
        aSTime  = Ta + Tb + Tz/2;
        bSTime = Tz/2;
        cSTime = Ta + Tz/2;
    otherwise
        error("Invalid quadrant in SVPWM");
end

== matlab function FullModel_Slow/PWM Generation/MATLAB Function3 ==
  data: Ta input; Tb input; Tc input; CCRA output; Ts input; CCRB output; CCRC output; ARR input
function [CCRA, CCRB, CCRC] = time2duty(Ta, Tb, Tc, Ts, ARR)
% This function converts switching times to CCR values for timers
% set in PWM Mode 3 - Center Aligned

dcA = Ta / Ts;
dcB = Tb / Ts;
dcC = Tc / Ts;

% CCRA / ARR = dcA;
CCRA = ARR * (1-dcA);
CCRB = ARR * (1-dcB);
CCRC = ARR * (1-dcC);
end

== matlab function FullModel_Slow/Hall Sensors/MATLAB Function ==
  settings: updateMethod=DISCRETE  sampleTime=1e-3
  data: angleRad input; H1 output; H2 output; H3 output; angleRad output
function [H1, H2, H3, angleRad] = angle2hall(angleRad)

HALL_DEGREES = pi/3;

% The LUT was built according to maxon catalogue page 67
% https://online.flippingbook.com/view/398826/67/#zoom=true

HALL_OUT_LUT_60 = [1,0,1;1,0,0;1,1,0;0,1,0;0,1,1;0,0,1];

% angleDeg = angleRad * (180/pi);
% angleRad = 2*pi - angleRad  ;

angleRad = angleRad * 8;
angleRad = mod(angleRad, 2*pi);

anglePosition = round(angleRad/HALL_DEGREES);

if anglePosition > 6
    anglePosition = 1;
end

if anglePosition < 1
    anglePosition = 1;
end

H1 = HALL_OUT_LUT_60(anglePosition,1);
H2 = HALL_OUT_LUT_60(anglePosition,2);
H3 = HALL_OUT_LUT_60(anglePosition,3);



end

== matlab function FullModel_Slow/AVG/MATLAB Function3 ==
  settings: updateMethod=DISCRETE
  data: in input; out output
function out = AVG(in)
N = 10;

persistent outSum

if isempty(outSum)
    outSum = 0;
end

outSum = outSum - outSum./N;
outSum = outSum + in ./N;

out = outSum;

== matlab function FullModel_Slow/Subsystem/Id//Iq Regulator1/MATLAB Function ==
  settings: updateMethod=DISCRETE
  data: P input; y output; I input; Ref input; x input
function y  = pidDiocan(P,I, Ref, x)
    
    persistent integral

    if isempty(integral)
        integral = 0;
    end

    error = Ref -x;
    y = error * P + integral * I;

    integral = integral + error;

== matlab function FullModel_Slow/Subsystem/Id//Iq Regulator1/MATLAB Function1 ==
  data: P input; y output; I input; Ref input; x input
function y  = pidDiocan(P,I, Ref, x)
    
    persistent integral

    if isempty(integral)
        integral = 0;
    end

    error = Ref - x;
    y = error * P + integral * I;

    integral = integral + error;

== matlab function FullModel_Slow/AVG/MATLAB Function4 ==
  settings: updateMethod=DISCRETE  sampleTime=1E-4
  data: in input; out output
function out = AVG(in)
N = 10;

persistent outSum

if isempty(outSum)
    outSum = 0;
end

outSum = outSum - outSum./N;
outSum = outSum + in ./N;

out = outSum;

== matlab function FullModel_Slow/Subsystem/MATLAB Function4 ==
  data: dq0 input; theta input; out output
function out = park2clarke(dq0,theta)
out = zeros(3, 1);
cosine = cos(theta);
sine = sin(theta);

% Q aligned
% out(1) = dq0(1) * sine + dq0(2) * cosine;
% out(2) = - dq0(1) * cosine + dq0(2) * sine;
% out(3) = 0;

% D aligned
out(1) = dq0(1) * cosine - dq0(2) * sine;
out(2) = dq0(1) * sine + dq0(2) * cosine;
out(3) = 0;
